simulink model "TransmissionPlant"  (R2026a)
settings: Solver=daessc
libraries: sdl_lib x24, fl_lib x19, nesl_utility x15
(part 2 of 2)

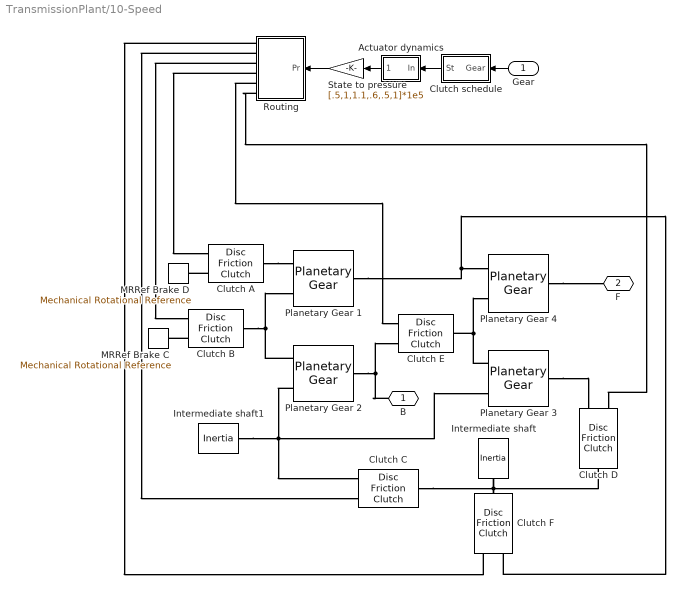
== system TransmissionPlant/10-Speed ==
  Gear : Inport
  Actuator dynamics : Subsystem  mask(First-order lag supporting vector signals){b=[1 1 1 1 1 1]*0.05, x_initial=ClutchSchedule{InitGear}}
      mask prompts: b "Filter time constant"; x_initial "Initial output"
      mask help: Models a lag of the form 1/(b*s+1) where s is the Laplace operator.
  Clutch schedule : Subsystem
  Clutch A : sdl_lib/Clutches/Disc Friction Clutch  geometry_model=1  r_eff=130 mm  d_o=150 mm  d_i=100 mm  nS=6  piston_area=1 m^2  unidirectional=0  friction_model=1  mu_w_vector=[0, 100, 1000] rad/s  temperature_TLU=[280, 300, 320] K  mu_static=0.35  mu_static_vector=[.4, .38, .36]  mu_coulomb=0.3  mu_coulomb_vector=[.3, .22, .19]  mu_coulomb_temp_vector=[.3, .28, .25]  mu_coulomb_matrix=[.34, .32, .3; .3, .28, .25; .25, .2, .15]  mu_interp_method=simscape.enum.interpolation.linear  mu_extrap_method=simscape.enum.extrapolation.linear  d_f=1  w_tol=0.001 rad/s  pressure_min=100 Pa  mu_visc=0 N*m/(rad/s)  initial_state_locked=1  thermal_mass=25 kJ/K  T_init=300 K
  Clutch B : sdl_lib/Clutches/Disc Friction Clutch  geometry_model=1  r_eff=130 mm  d_o=150 mm  d_i=100 mm  nS=10  piston_area=1 m^2  unidirectional=0  friction_model=1  mu_w_vector=[0, 100, 1000] rad/s  temperature_TLU=[280, 300, 320] K  mu_static=0.35  mu_static_vector=[.4, .38, .36]  mu_coulomb=0.3  mu_coulomb_vector=[.3, .22, .19]  mu_coulomb_temp_vector=[.3, .28, .25]  mu_coulomb_matrix=[.34, .32, .3; .3, .28, .25; .25, .2, .15]  mu_interp_method=simscape.enum.interpolation.linear  mu_extrap_method=simscape.enum.extrapolation.linear  d_f=1  w_tol=0.001 rad/s  pressure_min=100 Pa  mu_visc=0 N*m/(rad/s)  initial_state_locked=1  thermal_mass=25 kJ/K  T_init=300 K
  Clutch C : sdl_lib/Clutches/Disc Friction Clutch  geometry_model=1  r_eff=130 mm  d_o=150 mm  d_i=100 mm  nS=10  piston_area=1 m^2  unidirectional=0  friction_model=1  mu_w_vector=[0, 100, 1000] rad/s  temperature_TLU=[280, 300, 320] K  mu_static=0.35  mu_static_vector=[.4, .38, .36]  mu_coulomb=0.3  mu_coulomb_vector=[.3, .22, .19]  mu_coulomb_temp_vector=[.3, .28, .25]  mu_coulomb_matrix=[.34, .32, .3; .3, .28, .25; .25, .2, .15]  mu_interp_method=simscape.enum.interpolation.linear  mu_extrap_method=simscape.enum.extrapolation.linear  d_f=1  w_tol=0.001 rad/s  pressure_min=100 Pa  mu_visc=0 N*m/(rad/s)  initial_state_locked=0  thermal_mass=25 kJ/K  T_init=300 K
  Clutch D : sdl_lib/Clutches/Disc Friction Clutch  geometry_model=1  r_eff=130 mm  d_o=150 mm  d_i=100 mm  nS=12  piston_area=1 m^2  unidirectional=0  friction_model=1  mu_w_vector=[0, 100, 1000] rad/s  temperature_TLU=[280, 300, 320] K  mu_static=0.35  mu_static_vector=[.4, .38, .36]  mu_coulomb=0.3  mu_coulomb_vector=[.3, .22, .19]  mu_coulomb_temp_vector=[.3, .28, .25]  mu_coulomb_matrix=[.34, .32, .3; .3, .28, .25; .25, .2, .15]  mu_interp_method=simscape.enum.interpolation.linear  mu_extrap_method=simscape.enum.extrapolation.linear  d_f=1  w_tol=0.001 rad/s  pressure_min=100 Pa  mu_visc=0 N*m/(rad/s)  initial_state_locked=1  thermal_mass=25 kJ/K  T_init=300 K
  Clutch E : sdl_lib/Clutches/Disc Friction Clutch  geometry_model=1  r_eff=130 mm  d_o=150 mm  d_i=100 mm  nS=10  piston_area=1 m^2  unidirectional=0  friction_model=1  mu_w_vector=[0, 100, 1000] rad/s  temperature_TLU=[280, 300, 320] K  mu_static=0.35  mu_static_vector=[.4, .38, .36]  mu_coulomb=0.3  mu_coulomb_vector=[.3, .22, .19]  mu_coulomb_temp_vector=[.3, .28, .25]  mu_coulomb_matrix=[.34, .32, .3; .3, .28, .25; .25, .2, .15]  mu_interp_method=simscape.enum.interpolation.linear  mu_extrap_method=simscape.enum.extrapolation.linear  d_f=1  w_tol=0.001 rad/s  pressure_min=100 Pa  mu_visc=0 N*m/(rad/s)  initial_state_locked=0  thermal_mass=25 kJ/K  T_init=300 K
  Clutch F : sdl_lib/Clutches/Disc Friction Clutch  geometry_model=1  r_eff=130 mm  d_o=150 mm  d_i=100 mm  nS=8  piston_area=1 m^2  unidirectional=0  friction_model=1  mu_w_vector=[0, 100, 1000] rad/s  temperature_TLU=[280, 300, 320] K  mu_static=0.35  mu_static_vector=[.4, .38, .36]  mu_coulomb=0.3  mu_coulomb_vector=[.3, .22, .19]  mu_coulomb_temp_vector=[.3, .28, .25]  mu_coulomb_matrix=[.34, .32, .3; .3, .28, .25; .25, .2, .15]  mu_interp_method=simscape.enum.interpolation.linear  mu_extrap_method=simscape.enum.extrapolation.linear  d_f=1  w_tol=0.001 rad/s  pressure_min=100 Pa  mu_visc=0 N*m/(rad/s)  initial_state_locked=0  thermal_mass=25 kJ/K  T_init=300 K
  Intermediate shaft : fl_lib/Mechanical/Rotational Elements/Inertia  inertia=0.01 kg*m^2  num_ports=foundation.enum.numPorts2.one  w_specify=off  w_priority=High  w=0 rad/s  w_nominal_specify=off  w_nominal_value=1  w_nominal_unit=rad/s  t_specify=off  t_priority=High  t=0 N*m  t_nominal_specify=off  t_nominal_value=1  t_nominal_unit=N*m
  Intermediate shaft1 : fl_lib/Mechanical/Rotational Elements/Inertia  inertia=0.01 kg*m^2  num_ports=foundation.enum.numPorts2.one  w_specify=off  w_priority=High  w=0 rad/s  w_nominal_specify=off  w_nominal_value=1  w_nominal_unit=rad/s  t_specify=off  t_priority=High  t=0 N*m  t_nominal_specify=off  t_nominal_value=1  t_nominal_unit=N*m
  MRRef Brake C : fl_lib/Mechanical/Rotational Elements/Mechanical Rotational Reference
  MRRef Brake D : fl_lib/Mechanical/Rotational Elements/Mechanical Rotational Reference
  Planetary Gear 1 : sdl_lib/Gears/Planetary Gear  rs_ratio=92/44  friction_model=1  efficiency=[ 0.96 0.98 ]  temperature_TLU=[ 280 300 320 ] K  efficiency_sp_TLU=[ 0.95 0.9 0.85 ]  efficiency_rp_TLU=[ 0.95 0.9 0.85 ]  pwr_thr=[ 0.001 0.001 ] W  mu_visc=[ 0 0 ] N*m/(rad/s)  model_inertia=0  sun_inertia=1e-10 kg*m^2  ring_inertia=1e-10 kg*m^2  carrier_inertia=1e-10 kg*m^2  carrier_radius=0.01 m  planet_inertia=0.001 kg*m^2  planet_mass=1e-10 kg  thermal_mass=50 J/K  T_init=300 K
  Planetary Gear 2 : sdl_lib/Gears/Planetary Gear  rs_ratio=89/51  friction_model=1  efficiency=[ 0.96 0.98 ]  temperature_TLU=[ 280 300 320 ] K  efficiency_sp_TLU=[ 0.95 0.9 0.85 ]  efficiency_rp_TLU=[ 0.95 0.9 0.85 ]  pwr_thr=[ 0.001 0.001 ] W  mu_visc=[ 0 0 ] N*m/(rad/s)  model_inertia=0  sun_inertia=1e-10 kg*m^2  ring_inertia=1e-10 kg*m^2  carrier_inertia=1e-10 kg*m^2  carrier_radius=0.01 m  planet_inertia=0.001 kg*m^2  planet_mass=1e-10 kg  thermal_mass=50 J/K  T_init=300 K
  Planetary Gear 3 : sdl_lib/Gears/Planetary Gear  rs_ratio=101/63  friction_model=1  efficiency=[ 0.96 0.98 ]  temperature_TLU=[ 280 300 320 ] K  efficiency_sp_TLU=[ 0.95 0.9 0.85 ]  efficiency_rp_TLU=[ 0.95 0.9 0.85 ]  pwr_thr=[ 0.001 0.001 ] W  mu_visc=[ 0 0 ] N*m/(rad/s)  model_inertia=0  sun_inertia=1e-10 kg*m^2  ring_inertia=1e-10 kg*m^2  carrier_inertia=1e-10 kg*m^2  carrier_radius=0.01 m  planet_inertia=0.001 kg*m^2  planet_mass=1e-10 kg  thermal_mass=50 J/K  T_init=300 K
  Planetary Gear 4 : sdl_lib/Gears/Planetary Gear  rs_ratio=85/23  friction_model=1  efficiency=[ 0.96 0.98 ]  temperature_TLU=[ 280 300 320 ] K  efficiency_sp_TLU=[ 0.95 0.9 0.85 ]  efficiency_rp_TLU=[ 0.95 0.9 0.85 ]  pwr_thr=[ 0.001 0.001 ] W  mu_visc=[ 0 0 ] N*m/(rad/s)  model_inertia=0  sun_inertia=1e-10 kg*m^2  ring_inertia=1e-10 kg*m^2  carrier_inertia=1e-10 kg*m^2  carrier_radius=0.01 m  planet_inertia=0.001 kg*m^2  planet_mass=1e-10 kg  thermal_mass=50 J/K  T_init=300 K
  Routing : Subsystem
  State to pressure : Gain  Gain=[.5,1,1.1,.6,.5,1]*1e5
  B : PMIOPort  Side=Left
  F : PMIOPort  Port=2  Side=Right
  wires:
  Gear/1 -> Clutch schedule/1(Gear)
  Clutch schedule/1(St) -> Actuator dynamics/1(In)
  State to pressure/1 -> Routing/1(Pr)
  Actuator dynamics/1(Out) -> State to pressure/1
  connections:
  Clutch A/LConn2 -- MRRef Brake D/LConn1
  Clutch B/LConn2 -- MRRef Brake C/LConn1
  Planetary Gear 4/LConn1 -- F/RConn1
  B/RConn1 -- Planetary Gear 2/LConn1 -- Clutch E/LConn2
  Clutch A/RConn1 -- Planetary Gear 1/RConn1
  Clutch B/RConn1 -- Planetary Gear 1/RConn2 -- Planetary Gear 2/RConn2
  Planetary Gear 1/LConn1 -- Planetary Gear 4/RConn1 -- Clutch F/LConn2
  Planetary Gear 2/RConn1 -- Intermediate shaft1/LConn1 -- Planetary Gear 3/RConn2 -- Clutch C/LConn2
  Planetary Gear 3/RConn1 -- Clutch E/RConn1 -- Planetary Gear 4/RConn2
  Planetary Gear 3/LConn1 -- Clutch D/LConn2
  Clutch F/RConn1 -- Clutch C/RConn1 -- Intermediate shaft/LConn1 -- Clutch D/RConn1
  Routing/RConn1 -- Clutch F/LConn1
  Routing/RConn2 -- Clutch C/LConn1
  Routing/RConn3 -- Clutch B/LConn1
  Routing/RConn4 -- Clutch A/LConn1
  Routing/RConn5 -- Clutch E/LConn1
  Routing/RConn6 -- Clutch D/LConn1

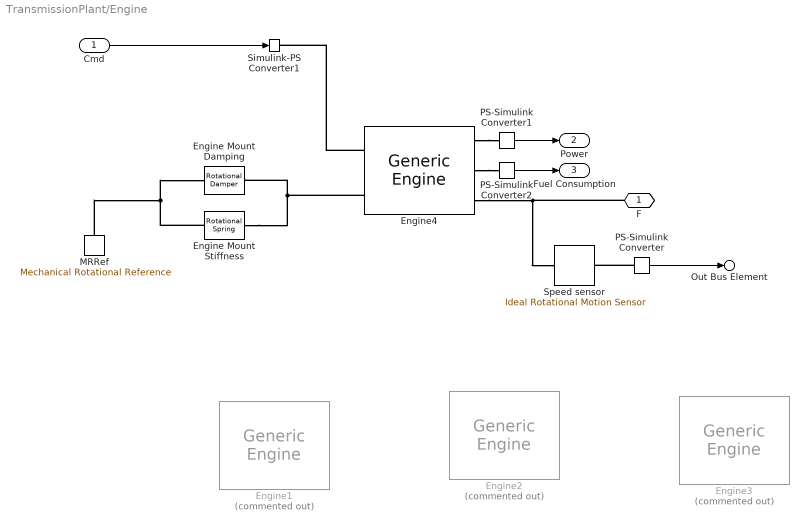
== system TransmissionPlant/Engine ==
  Cmd : Inport
  Engine Mount Damping : fl_lib/Mechanical/Rotational Elements/Rotational Damper  D=10000 N*m/rpm  w_specify=on  w_priority=High  w=0 rad/s  w_nominal_specify=off  w_nominal_value=1  w_nominal_unit=rad/s  t_specify=off  t_priority=High  t=0 N*m  t_nominal_specify=off  t_nominal_value=1  t_nominal_unit=N*m
      settings: AttributesFormatString=|
      | %<D>
      | %<D_unit>
  Engine Mount Stiffness : fl_lib/Mechanical/Rotational Elements/Rotational Spring  spr_rate=10 N*m/rad  w_specify=on  w_priority=High  w=0 rad/s  w_nominal_specify=off  w_nominal_value=1  w_nominal_unit=rad/s  t_specify=off  t_priority=High  t=0 N*m  t_nominal_specify=off  t_nominal_value=1  t_nominal_unit=N*m  phi_specify=off  phi_priority=High  phi=0 rad  phi_nominal_specify=off  phi_nominal_value=1  phi_nominal_unit=rad
      settings: AttributesFormatString=|
      | %<spr_rate>
      | %<spr_rate_unit>
  Engine1 : sdl_lib/Engines & Motors/Generic Engine  Commented=on  input_type=sdl.enum.GenericEngineInputType.NormalizedThrottle  model_parameterization=1  engine_type=1  Trq_max=380 N*m  w_Trq_max=4300 rpm  P_max=100 kW  w_P_max=5500 rpm  w_max=7500 rpm  w_min=200 rpm  w_tab=[ 500 1000 2e+3 3e+3 4e+3 5e+3 6e+3 7e+3 ] rpm  trq_tab=[ 380 380 380 380 350 280 200 80 ] N*m  pwr_tab=[ 2e+4 4e+4 7.8e+4 1.2e+5 1.45e+5 1.48e+5 1.25e+5 6e+4 ] W  interp_method=simscape.enum.interpolation.linear  w_thr=20 rpm  model_inertia=1  inertia=0.2 kg*m^2  initial_velocity=800 rpm  model_time_constant=1  time_constant=0.2 s  initial_normalized_throttle=0  fc_model=sdl.enum.fuel_consumption_model.FuelSpeedTorque  fc_per_rev=25 mg/rev  fc_w_tab=[ 1000 2e+3 3e+3 4e+3 5e+3 6e+3 ] rpm  fc_trq_tab=[ 0 80 160 200 240 320 360 400 ] N*m  fc_tab=[ 0.5 0.9 1.4 1.6 1.9 2.7 3.4 4.4; 1 1.7 2.7 3.1 3.6 5 6 7.4; 1.4 2.7 4 4.8 5.6 7.5 8.5 10.5; 2 3.6 5.8 6.7 8 10.4 11.7 13.3; 2.5 4.8 7.9 9.4 10.8 14 16.2 18.6; 3.1 6 10.3 11.9 13.8 18.4 22 26.5 ] g/s  bmep_tab=[ 0 250 500 625 750 1000 1.15e+3 1.25e+3 ] kPa  bsfc_tab=[ 410 380 300 280 270 290 320 380; 410 370 290 270 260 270 285 320; 415 380 290 275 265 270 270 300; 420 390 310 290 285 280 280 285; 430 410 340 320 310 300 310 320; 450 430 370 340 330 330 350 380 ] g/hr/kW  fc_interp_method=simscape.enum.interpolation.linear  displaced_volume=400 cm^3  rev_per_cycle=2  idle_speed=1  idle_speed_reference=800 rpm  tau_controller=0.1 s  idle_w_thr=1 rpm  redline=true  redline_speed=6800 rpm  tau_redline=1 s  redline_w_thr=1 rpm
      settings: AttributesFormatString=%<initial_velocity> [%<initial_velocity_unit>]
  Engine2 : sdl_lib/Engines & Motors/Generic Engine  Commented=on  PartSpecification="{\"CollectionId\":\"MW.SimscapeDriveline\",\"CollectionVersion\":\"1.0.0\",\"DatasetId\":\"Generic Engine|325 hp Engine Gasoline: Tier 3|simscape.driveline.genericEngine\",\"DisplayName\":\"Generic Engine:325 hp Engine Gasoline: Tier 3\"}"  input_type=sdl.enum.GenericEngineInputType.NormalizedThrottle  model_parameterization=sdl.enum.engineParameterization.torque  engine_type=sdl.enum.engineType.SI  Trq_max=380 % Parameter not set N*m  w_Trq_max=4300 % Parameter not set rpm  P_max=230 % Parameter not set kW  w_P_max=6858 % Parameter not set rpm  w_max=7000 % Parameter not set rpm  w_min=500 % Parameter not set rpm  w_tab=[1000;1501;1751;2000;3000;4250;5750;6037.5] % From weblink database rpm  trq_tab=[230.06;350.03;416.41;460.978;508.432;488.094;402.678;345.153] % From weblink database N*m  pwr_tab=[10, 30, 70, 110, 165, 190, 220, 230] % Parameter not set kW  interp_method=simscape.enum.interpolation.smooth  w_thr=100 % Library default rpm  model_inertia=sdl.enum.model_inertia.off  inertia=1 % Parameter not set kg*m^2  initial_velocity=800 % Parameter not set rpm  model_time_constant=sdl.enum.lagOffOn.off  time_constant=0.2 % Parameter not set s  initial_normalized_throttle=0 % Parameter not set  fc_model=sdl.enum.fuel_consumption_model.FuelSpeedTorque  fc_per_rev=25 % Parameter not set mg/rev  fc_w_tab=[0.01 300.417 600.833 1001.167 1251.115 1501.094 1751.059 2001.1 2251.118 2501.029 2751 3001.972 3502.245 4002.16 4501.969 5013.389 5496.816 5910.908 6325] % From weblink database rpm  fc_trq_tab=[25.219 55.538 80.156 104.375 117.652 144.49 178.614 199.144 225.9 250.615 280.405 315.274 344.012 376.651 405.257 438.688 469.19 491.928 512.891 533.853] % From weblink database N*m  fc_tab=[0.083 0.07 0.099 0.157 0.197 0.294 0.465 0.581 0.733 0.847 0.927 0.915 0.823 0.662 0.507 0.317 0.121 0.01 0.01 0.01;0.144 0.182 0.268 0.356 0.409 0.537 0.747 0.892 1.089 1.26 1.418 1.476 1.444 1.371 1.318 1.284 1.271 1.268 1.268 1.269;0.204 0.297 0.439 0.553 0.622 0.781 1.033 1.206 1.442 1.669 1.906 2.033 2.063 2.084 2.133 2.25 2.42 2.575 2.731 2.893;0.315 0.474 0.631 0.815 0.915 1.114 1.432 1.638 1.907 2.189 2.536 2.752 2.885 3.058 3.239 3.532 3.942 4.313 4.682 5.062;0.375 0.605 0.801 1.005 1.111 1.33 1.704 1.914 2.212 2.49 2.88 3.17 3.403 3.693 3.955 4.329 4.887 5.397 5.901 6.416;0.442 0.725 0.966 1.194 1.319 1.58 1.955 2.18 2.463 2.767 3.161 3.565 3.929 4.346 4.69 5.13 5.833 6.482 7.117 7.764;0.515 0.865 1.126 1.387 1.538 1.836 2.226 2.459 2.751 3.077 3.467 3.973 4.474 5.016 5.445 5.95 6.788 7.569 8.326 9.099;0.614 1.009 1.279 1.58 1.753 2.095 2.514 2.765 3.093 3.436 3.845 4.405 5.024 5.695 6.204 6.831 7.765 8.656 9.521 10.407;0.729 1.156 1.455 1.794 1.985 2.366 2.819 3.098 3.472 3.839 4.275 4.847 5.521 6.331 6.961 7.851 8.794 9.729 10.689 11.668;0.844 1.301 1.643 2.025 2.235 2.649 3.138 3.447 3.868 4.27 4.727 5.336 6.061 6.939 7.634 8.773 9.686 10.759 11.821 12.857;0.974 1.456 1.844 2.26 2.487 2.936 3.473 3.813 4.27 4.71 5.197 5.865 6.557 7.562 8.42 9.477 10.34 11.729 12.888 13.941;1.116 1.631 2.065 2.5 2.742 3.231 3.827 4.193 4.675 5.132 5.67 6.4 7.135 8.235 9.263 9.923 10.776 12.604 13.823 14.901;1.348 1.962 2.472 2.982 3.265 3.844 4.568 4.99 5.494 5.982 6.627 7.523 8.433 9.572 10.47 11.259 12.038 12.938 14.583 16.301;1.581 2.321 2.919 3.492 3.809 4.475 5.31 5.762 6.337 6.921 7.762 8.873 9.933 11.065 11.831 13.006 14.082 15.187 16.454 17.83;1.909 2.716 3.377 4.035 4.397 5.139 6.086 6.635 7.339 8.038 9.13 10.479 11.735 13.201 14.563 16.257 17.398 18.298 19.183 20.103;2.232 3.084 3.824 4.577 4.997 5.859 7.005 7.727 8.714 9.714 11.061 12.755 14.229 16.286 18.734 20.266 21.207 21.896 22.545 23.203;2.48 3.426 4.246 5.096 5.576 6.581 7.98 8.9 10.19 11.491 13.205 15.377 17.023 19.824 22.002 23.679 24.736 25.425 26.039 26.647;2.653 3.705 4.608 5.548 6.084 7.222 8.859 9.957 11.505 13.063 15.092 17.629 19.777 22.493 24.574 26.43 27.67 28.454 29.131 29.794;2.811 3.977 4.968 6.003 6.598 7.873 9.753 11.029 12.833 14.646 17.001 19.966 22.462 25.107 27.137 29.13 30.565 31.475 32.251 33.004] % From weblink database g/s  bmep_tab=[0, 250, 500, 625, 750, 1000, 1150, 1250] % Parameter not set kPa  bsfc_tab=[410, 380, 300, 280, 270, 290, 320, 380; 410, 370, 290, 270, 260, 270, 285, 320; 415, 380, 290, 275, 265, 270, 270, 300; 420, 390, 310, 290, 285, 280, 280, 285; 430, 410, 340, 320, 310, 300, 310, 320; 450, 430, 370, 340, 330, 330, 350, 380] % Parameter not set g/(hr*kW)  fc_interp_method=simscape.enum.interpolation.linear  displaced_volume=400 % Parameter not set cm^3  rev_per_cycle=2 % Parameter not set  idle_speed=true  idle_speed_reference=800 rpm  tau_controller=0.1 s  idle_w_thr=1 rpm  redline=true  redline_speed=5000 % Parameter not set rpm  tau_redline=0.1 s  redline_w_thr=1 % Parameter not set rpm
      settings: AttributesFormatString=Generic Engine:325 hp Engine Gasoline: Tier 3
  Engine3 : sdl_lib/Engines & Motors/Generic Engine  Commented=on  PartSpecification="{\"CollectionId\":\"MW.SimscapeDriveline\",\"CollectionVersion\":\"1.0.0\",\"DatasetId\":\"Generic Engine|155 hp Engine Gasoline: Tier 2|simscape.driveline.genericEngine\",\"DisplayName\":\"Generic Engine:155 hp Engine Gasoline: Tier 2\"}"  input_type=sdl.enum.GenericEngineInputType.NormalizedThrottle  model_parameterization=sdl.enum.engineParameterization.polynomial  engine_type=sdl.enum.engineType.SI  Trq_max=380 % Parameter not set N*m  w_Trq_max=4300 % Parameter not set rpm  P_max=230 % Parameter not set kW  w_P_max=6858 % Parameter not set rpm  w_max=7000 % Parameter not set rpm  w_min=500 % Parameter not set rpm  w_tab=[1012.176;1202.696;1301.407;1499.571;1699.486;1900.487;2000.333;2199.867;2400.438;2700.87;2997.792;3300.957;3400.557;3801.205;4100.143;4482.885;6000;6250;6562.5] % From weblink database rpm  trq_tab=[138.688;150.113;153.022;164.067;167.811;183.362;187.874;188.469;182.602;188.231;201.838;199.89;197.399;196.929;200.098;195.305;184;160;130] % From weblink database N*m  pwr_tab=[10, 30, 70, 110, 165, 190, 220, 230] % Parameter not set kW  interp_method=simscape.enum.interpolation.smooth  w_thr=100 % Library default rpm  model_inertia=sdl.enum.model_inertia.off  inertia=1 % Parameter not set kg*m^2  initial_velocity=800 % Parameter not set rpm  model_time_constant=sdl.enum.lagOffOn.off  time_constant=0.2 % Parameter not set s  initial_normalized_throttle=0 % Parameter not set  fc_model=sdl.enum.fuel_consumption_model.FuelSpeedTorque  fc_per_rev=25 % Parameter not set mg/rev  fc_w_tab=[0.01 370.5 741.001 847.204 987.232 1249.539 1497.588 1640.802 1746.865 1869.12 1998.314 2495.794 2995.594 3494.811 3994.431 4494.065 4997.033 5500 6187.5 6875] % From weblink database rpm  fc_trq_tab=[0.519 9.925 19.919 29.858 39.992 49.571 59.937 69.931 80.019 89.98 99.967 110.094 119.924 129.762 139.529 150.227 160.094 169.961 181.674 188.912 196.15 204.039 211.929] % From weblink database N*m  fc_tab=[0.03 0.049 0.069 0.084 0.09 0.088 0.083 0.08 0.082 0.091 0.108 0.135 0.175 0.232 0.304 0.393 0.472 0.547 0.629 0.678 0.725 0.775 0.825;0.074 0.096 0.13 0.168 0.186 0.202 0.219 0.238 0.262 0.292 0.33 0.379 0.435 0.503 0.588 0.699 0.806 0.91 1.033 1.107 1.181 1.262 1.343;0.12 0.145 0.192 0.247 0.28 0.316 0.356 0.396 0.44 0.494 0.552 0.621 0.698 0.778 0.874 1.001 1.135 1.274 1.436 1.536 1.637 1.749 1.863;0.133 0.161 0.211 0.267 0.307 0.349 0.395 0.441 0.492 0.551 0.616 0.69 0.775 0.86 0.957 1.086 1.228 1.379 1.551 1.659 1.768 1.889 2.012;0.15 0.184 0.239 0.295 0.344 0.392 0.447 0.502 0.56 0.627 0.7 0.781 0.876 0.968 1.067 1.197 1.349 1.517 1.704 1.82 1.94 2.073 2.208;0.185 0.234 0.296 0.358 0.425 0.479 0.549 0.615 0.689 0.766 0.859 0.951 1.063 1.177 1.278 1.403 1.572 1.774 1.987 2.124 2.264 2.42 2.576;0.219 0.283 0.355 0.43 0.503 0.574 0.66 0.738 0.824 0.913 1.008 1.108 1.23 1.39 1.488 1.6 1.775 2.002 2.254 2.414 2.574 2.748 2.921;0.241 0.312 0.392 0.472 0.55 0.63 0.72 0.811 0.904 1.002 1.099 1.2 1.321 1.486 1.601 1.72 1.892 2.121 2.409 2.584 2.755 2.938 3.119;0.257 0.333 0.419 0.504 0.586 0.671 0.764 0.865 0.964 1.069 1.169 1.269 1.389 1.552 1.679 1.809 1.979 2.202 2.524 2.711 2.89 3.079 3.265;0.276 0.357 0.451 0.54 0.628 0.718 0.814 0.926 1.035 1.147 1.251 1.352 1.468 1.624 1.763 1.91 2.08 2.288 2.657 2.858 3.046 3.241 3.432;0.297 0.382 0.484 0.577 0.672 0.769 0.867 0.991 1.109 1.229 1.34 1.441 1.555 1.702 1.849 2.017 2.189 2.378 2.802 3.016 3.212 3.413 3.609;0.377 0.483 0.598 0.717 0.844 0.971 1.116 1.253 1.396 1.543 1.69 1.831 1.983 2.11 2.269 2.454 2.679 2.993 3.49 3.68 3.862 4.068 4.281;0.483 0.6 0.733 0.878 1.034 1.195 1.371 1.538 1.706 1.869 2.031 2.217 2.39 2.561 2.732 2.935 3.186 3.519 4.011 4.272 4.506 4.764 5.013;0.579 0.725 0.888 1.074 1.271 1.456 1.646 1.845 2.041 2.234 2.438 2.651 2.861 3.047 3.228 3.44 3.687 4.019 4.608 4.978 5.291 5.565 5.835;0.718 0.885 1.077 1.302 1.55 1.758 1.989 2.19 2.396 2.612 2.838 3.077 3.311 3.538 3.765 4.002 4.277 4.651 5.258 5.633 5.992 6.399 6.838;0.852 1.067 1.296 1.52 1.753 2.009 2.282 2.537 2.784 3.024 3.262 3.525 3.779 4.029 4.294 4.637 4.998 5.427 6.205 6.684 7.15 7.648 8.145;1.017 1.263 1.52 1.77 2.031 2.296 2.598 2.896 3.197 3.49 3.771 4.042 4.303 4.584 4.919 5.406 5.996 6.692 7.594 8.118 8.619 9.148 9.669;1.185 1.463 1.755 2.029 2.314 2.597 2.923 3.257 3.608 3.964 4.312 4.608 4.903 5.241 5.654 6.269 7.123 8.094 9.198 9.724 10.223 10.765 11.309;1.401 1.709 2.034 2.354 2.683 3.003 3.365 3.734 4.126 4.527 4.939 5.373 5.833 6.366 7.002 7.855 8.784 9.786 10.969 11.655 12.316 13.016 13.709;1.604 1.946 2.308 2.668 3.037 3.391 3.786 4.184 4.613 5.075 5.591 6.186 6.846 7.595 8.426 9.43 10.423 11.462 12.742 13.545 14.352 15.232 16.112] % From weblink database g/s  bmep_tab=[0, 250, 500, 625, 750, 1000, 1150, 1250] % Parameter not set kPa  bsfc_tab=[410, 380, 300, 280, 270, 290, 320, 380; 410, 370, 290, 270, 260, 270, 285, 320; 415, 380, 290, 275, 265, 270, 270, 300; 420, 390, 310, 290, 285, 280, 280, 285; 430, 410, 340, 320, 310, 300, 310, 320; 450, 430, 370, 340, 330, 330, 350, 380] % Parameter not set g/(hr*kW)  fc_interp_method=simscape.enum.interpolation.linear  displaced_volume=400 % Parameter not set cm^3  rev_per_cycle=2 % Parameter not set  idle_speed=true  idle_speed_reference=1000 % Parameter not set rpm  tau_controller=1 % Parameter not set s  idle_w_thr=1 % Parameter not set rpm  redline=true  redline_speed=5000 % Parameter not set rpm  tau_redline=1 % Parameter not set s  redline_w_thr=1 % Parameter not set rpm
      settings: AttributesFormatString=Generic Engine:155 hp Engine Gasoline: Tier 2
  Engine4 : sdl_lib/Engines & Motors/Generic Engine  input_type=sdl.enum.GenericEngineInputType.NormalizedThrottle  model_parameterization=1  engine_type=1  Trq_max=380 N*m  w_Trq_max=4300 rpm  P_max=100 kW  w_P_max=5500 rpm  w_max=7500 rpm  w_min=200 rpm  w_tab=[ 500 1000 2e+3 3e+3 4e+3 5e+3 6e+3 7e+3 ] rpm  trq_tab=[ 380 380 380 380 350 280 200 80 ] N*m  pwr_tab=[ 2e+4 4e+4 7.8e+4 1.2e+5 1.45e+5 1.48e+5 1.25e+5 6e+4 ] W  interp_method=simscape.enum.interpolation.linear  w_thr=20 rpm  model_inertia=1  inertia=0.2 kg*m^2  initial_velocity=800 rpm  model_time_constant=1  time_constant=0.2 s  initial_normalized_throttle=0  fc_model=sdl.enum.fuel_consumption_model.FuelSpeedTorque  fc_per_rev=25 mg/rev  fc_w_tab=[ 1000 2e+3 3e+3 4e+3 5e+3 6e+3 ] rpm  fc_trq_tab=[ 0 80 160 200 240 320 360 400 ] N*m  fc_tab=[ 0.5 0.9 1.4 1.6 1.9 2.7 3.4 4.4; 1 1.7 2.7 3.1 3.6 5 6 7.4; 1.4 2.7 4 4.8 5.6 7.5 8.5 10.5; 2 3.6 5.8 6.7 8 10.4 11.7 13.3; 2.5 4.8 7.9 9.4 10.8 14 16.2 18.6; 3.1 6 10.3 11.9 13.8 18.4 22 26.5 ] g/s  bmep_tab=[ 0 250 500 625 750 1000 1.15e+3 1.25e+3 ] kPa  bsfc_tab=[ 410 380 300 280 270 290 320 380; 410 370 290 270 260 270 285 320; 415 380 290 275 265 270 270 300; 420 390 310 290 285 280 280 285; 430 410 340 320 310 300 310 320; 450 430 370 340 330 330 350 380 ] g/hr/kW  fc_interp_method=simscape.enum.interpolation.linear  displaced_volume=400 cm^3  rev_per_cycle=2  idle_speed=false  idle_speed_reference=800 rpm  tau_controller=0.1 s  idle_w_thr=1 rpm  redline=false  redline_speed=6800 rpm  tau_redline=1 s  redline_w_thr=1 rpm
      settings: AttributesFormatString=%<initial_velocity> [%<initial_velocity_unit>]
  MRRef : fl_lib/Mechanical/Rotational Elements/Mechanical Rotational Reference
  PS-Simulink Converter : nesl_utility/PS-Simulink Converter  PhysicalDomain=network_engine_domain  SubClassName=ps_output  LeftPortType=input  RightPortType=output  PseudoPeriodic=off  Frequencies=[]  VectorFormat=inherit  Unit=rpm  AffineConversion=off
  PS-Simulink Converter1 : nesl_utility/PS-Simulink Converter  PhysicalDomain=network_engine_domain  SubClassName=ps_output  LeftPortType=input  RightPortType=output  PseudoPeriodic=off  Frequencies=[]  VectorFormat=inherit  Unit=inherit  AffineConversion=off
  PS-Simulink Converter2 : nesl_utility/PS-Simulink Converter  PhysicalDomain=network_engine_domain  SubClassName=ps_output  LeftPortType=input  RightPortType=output  PseudoPeriodic=off  Frequencies=[]  VectorFormat=inherit  Unit=inherit  AffineConversion=off
  Simulink-PS Converter1 : nesl_utility/Simulink-PS Converter  PhysicalDomain=network_engine_domain  SubClassName=ps_input  LeftPortType=input  RightPortType=output  PseudoPeriodic=off  Frequencies=[]  NoiseDistribution=none  NoiseParameters=[]  Unit=1  AffineConversion=off  FilteringAndDerivatives=provide  SimscapeFilterOrder=1  InputFilterTimeConstant=0.001  UdotUserProvided=0
  Speed sensor : fl_lib/Mechanical/Mechanical Sensors/Ideal Rotational Motion Sensor  reference=foundation.enum.MeasurementReference.absolute  acceleration_port=false  velocity_port=true  position_port=false  wrap_angle=simscape.enum.onoff.off  offset=0 rad
  F : PMIOPort  Side=Left
  Out Bus Element : Outport  PortName=Info  Element=EngSpd
  Power : Outport  Port=2
  Fuel Consumption : Outport  Port=3
  wires:
  PS-Simulink Converter/1 -> Out Bus Element/1
  Cmd/1 -> Simulink-PS Converter1/1
  PS-Simulink Converter1/1 -> Power/1
  PS-Simulink Converter2/1 -> Fuel Consumption/1
  connections:
  Engine Mount Stiffness/RConn1 -- Engine4/LConn2 -- Engine Mount Damping/RConn1
  F/RConn1 -- Engine4/RConn3 -- Speed sensor/LConn1
  Engine Mount Stiffness/LConn1 -- MRRef/LConn1 -- Engine Mount Damping/LConn1
  PS-Simulink Converter/LConn1 -- Speed sensor/RConn1
  Engine4/LConn1 -- Simulink-PS Converter1/RConn1
  Engine4/RConn1 -- PS-Simulink Converter1/LConn1
  Engine4/RConn2 -- PS-Simulink Converter2/LConn1

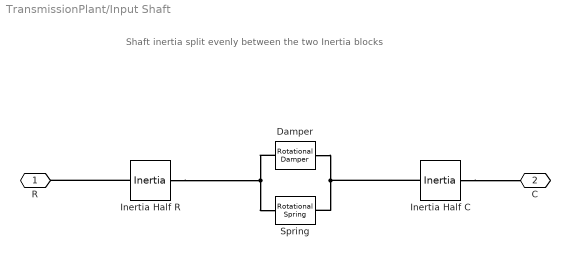
== system TransmissionPlant/Input Shaft ==
  note: Shaft inertia split evenly between the two Inertia blocks
  Damper : fl_lib/Mechanical/Rotational Elements/Rotational Damper  D=10000 N*m/rpm  w_specify=off  w_priority=High  w=0 rad/s  w_nominal_specify=off  w_nominal_value=1  w_nominal_unit=rad/s  t_specify=on  t_priority=High  t=0 N*m  t_nominal_specify=off  t_nominal_value=1  t_nominal_unit=N*m
      settings: AttributesFormatString=|
      | %<D>
      | %<D_unit>
  Inertia Half C : fl_lib/Mechanical/Rotational Elements/Inertia  inertia=0.0015 kg*m^2  num_ports=foundation.enum.numPorts2.two  w_specify=on  w_priority=High  w=800 rpm  w_nominal_specify=off  w_nominal_value=1  w_nominal_unit=rad/s  t_specify=off  t_priority=High  t=0 N*m  t_nominal_specify=off  t_nominal_value=1  t_nominal_unit=N*m
      settings: AttributesFormatString=|
      | %<inertia> %<inertia_unit>
      | %<w> [%<w_unit>]
      | Priority: %<w_priority>
  Inertia Half R : fl_lib/Mechanical/Rotational Elements/Inertia  inertia=0.0015 kg*m^2  num_ports=foundation.enum.numPorts2.two  w_specify=on  w_priority=High  w=800 rpm  w_nominal_specify=off  w_nominal_value=1  w_nominal_unit=rad/s  t_specify=off  t_priority=High  t=0 N*m  t_nominal_specify=off  t_nominal_value=1  t_nominal_unit=N*m
      settings: AttributesFormatString=|
      | %<inertia> %<inertia_unit>
      | %<w> [%<w_unit>]
      | Priority: %<w_priority>
  Spring : fl_lib/Mechanical/Rotational Elements/Rotational Spring  spr_rate=10 N*m/rad  w_specify=off  w_priority=High  w=0 rad/s  w_nominal_specify=off  w_nominal_value=1  w_nominal_unit=rad/s  t_specify=on  t_priority=High  t=0 N*m  t_nominal_specify=off  t_nominal_value=1  t_nominal_unit=N*m  phi_specify=off  phi_priority=High  phi=0 rad  phi_nominal_specify=off  phi_nominal_value=1  phi_nominal_unit=rad
      settings: AttributesFormatString=|
      | %<spr_rate>
      | %<spr_rate_unit>
  R : PMIOPort  Side=Left
  C : PMIOPort  Port=2  Side=Right
  connections:
  Damper/RConn1 -- Inertia Half C/LConn1 -- Spring/RConn1
  Damper/LConn1 -- Inertia Half R/RConn1 -- Spring/LConn1
  Inertia Half C/RConn1 -- C/RConn1
  Inertia Half R/LConn1 -- R/RConn1

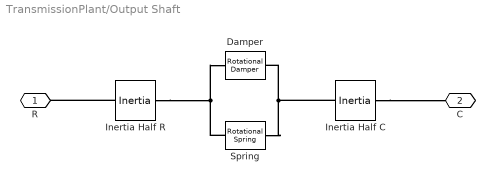
== system TransmissionPlant/Output Shaft ==
  Damper : fl_lib/Mechanical/Rotational Elements/Rotational Damper  D=20000 N*m/rpm  w_specify=off  w_priority=High  w=0 rad/s  w_nominal_specify=off  w_nominal_value=1  w_nominal_unit=rad/s  t_specify=off  t_priority=High  t=0 N*m  t_nominal_specify=off  t_nominal_value=1  t_nominal_unit=N*m
      settings: AttributesFormatString=|
      | %<D>
      | %<D_unit>
  "Inertia Half C " : fl_lib/Mechanical/Rotational Elements/Inertia  inertia=0.0001 kg*m^2  num_ports=foundation.enum.numPorts2.two  w_specify=on  w_priority=High  w=0 rad/s  w_nominal_specify=off  w_nominal_value=1  w_nominal_unit=rad/s  t_specify=off  t_priority=High  t=0 N*m  t_nominal_specify=off  t_nominal_value=1  t_nominal_unit=N*m
      settings: AttributesFormatString=|
      | %<inertia> %<inertia_unit>
      | %<w> [%<w_unit>]
      | Priority: %<w_priority>
  Inertia Half R : fl_lib/Mechanical/Rotational Elements/Inertia  inertia=0.0001 kg*m^2  num_ports=foundation.enum.numPorts2.two  w_specify=on  w_priority=High  w=0 rad/s  w_nominal_specify=off  w_nominal_value=1  w_nominal_unit=rad/s  t_specify=off  t_priority=High  t=0 N*m  t_nominal_specify=off  t_nominal_value=1  t_nominal_unit=N*m
      settings: AttributesFormatString=|
      | %<inertia> %<inertia_unit>
      | %<w> [%<w_unit>]
      | Priority: %<w_priority>
  Spring : fl_lib/Mechanical/Rotational Elements/Rotational Spring  spr_rate=10 N*m/rad  w_specify=off  w_priority=High  w=0 rad/s  w_nominal_specify=off  w_nominal_value=1  w_nominal_unit=rad/s  t_specify=off  t_priority=High  t=0 N*m  t_nominal_specify=off  t_nominal_value=1  t_nominal_unit=N*m  phi_specify=off  phi_priority=High  phi=0 rad  phi_nominal_specify=off  phi_nominal_value=1  phi_nominal_unit=rad
      settings: AttributesFormatString=|
      | %<spr_rate>
      | %<spr_rate_unit>
  R : PMIOPort  Side=Left
  C : PMIOPort  Port=2  Side=Right
  connections:
  Spring/RConn1 -- "Inertia Half C "/LConn1 -- Damper/RConn1
  Spring/LConn1 -- Inertia Half R/RConn1 -- Damper/LConn1
  Inertia Half R/LConn1 -- R/RConn1
  "Inertia Half C "/RConn1 -- C/RConn1

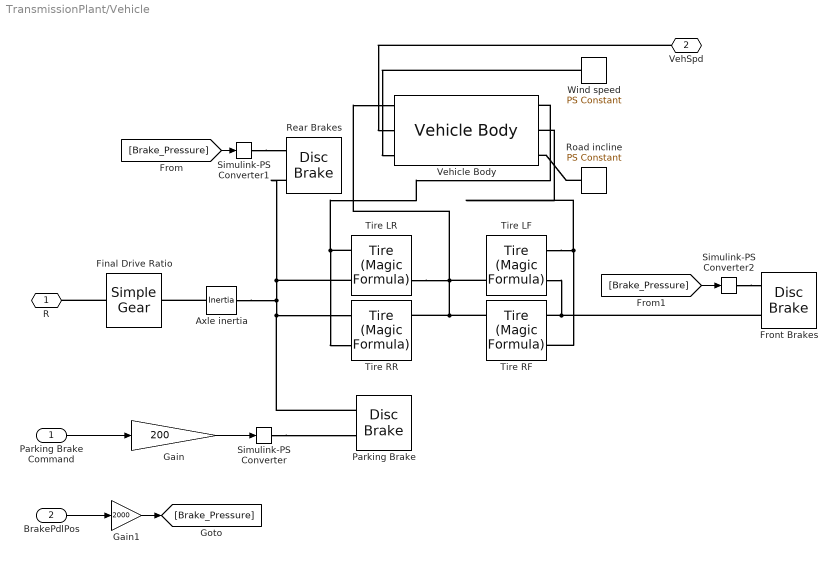
== system TransmissionPlant/Vehicle ==
  Parking Brake Command : Inport
  BrakePdlPos : Inport  Port=2
  Axle inertia : fl_lib/Mechanical/Rotational Elements/Inertia  inertia=0.01 kg*m^2  num_ports=foundation.enum.numPorts2.two  w_specify=on  w_priority=None  w=0 rad/s  w_nominal_specify=off  w_nominal_value=1  w_nominal_unit=rad/s  t_specify=off  t_priority=High  t=0 N*m  t_nominal_specify=off  t_nominal_value=1  t_nominal_unit=N*m
      settings: AttributesFormatString=Priority: %<w_priority>
  Final Drive Ratio : sdl_lib/Gears/Simple Gear  ratio=3.7  rotation_direction=sdl.enum.shaftOutputDirection.same  friction_model=2  T_noload=0.1 N*m  T_nom=5 N*m  efficiency_nom=0.8  efficiency=0.95  temperature_TLU=[ 280 300 320 ] K  load_TLU=[ 1 5 10 ] N*m  efficiency_TLU=[ 0.95 0.9 0.85 ]  efficiency_TLU2=[ 0.85 0.8 0.75; 0.95 0.9 0.85; 0.85 0.8 0.7 ]  w_thr=0.01 rad/s  pwr_thr=1 W  enable_backlash=false  hardstop_model=simscape.enum.hardstop.smooth  backlash_distance=1e-3 mm  r_base=0.1 m  transition=1e-4 mm  backlash_stiffness=1e7 N/m  backlash_damping=1e6 N*s/m  coeff_rest=0  v_tol=0.001 m/s  f_tol=0 N  tau=0.1 s  mu_visc=[0 0] N*m/(rad/s)  thermal_mass=50 J/K  temperature_specify=off  temperature_priority=High  temperature=300 K  temperature_nominal_specify=off  temperature_nominal_value=1  temperature_nominal_unit=K  x_backlash_specify=off  x_backlash_priority=None  x_backlash=0 mm  x_backlash_nominal_specify=off  x_backlash_nominal_value=1  x_backlash_nominal_unit=mm  f_hardstop_specify=off  f_hardstop_priority=None  f_hardstop=0 N  f_hardstop_nominal_specify=off  f_hardstop_nominal_value=1  f_hardstop_nominal_unit=N  v_backlash_specify=off  v_backlash_priority=None  v_backlash=0 m/s  v_backlash_nominal_specify=off  v_backlash_nominal_value=1  v_backlash_nominal_unit=m/s
      settings: AttributesFormatString=Reduction ratio %<ratio>
  Front Brakes : sdl_lib/Brakes & Detents/Rotational/Disc Brake  r_mean=150 mm  bore=10 mm  n_pads=2  thermal_port=simscape.enum.thermaleffects.omit  mu_static=0.9  mu_coulomb=0.7  temperature_TLU=[280, 300, 320] K  mu_static_TLU=[.9, .8, .7]  mu_coulomb_TLU=[.8, .7, .6]  brkwy_vel=0.1 rad/s  visc_coef=0 N*m*s/rad  thermal_mass=50 kJ/K  temperature_specify=off  temperature_priority=High  temperature=300 K  temperature_nominal_specify=off  temperature_nominal_value=1  temperature_nominal_unit=K
  Gain : Gain  Gain=200  OutDataTypeStr=double
  Gain1 : Gain  Gain=2000
  Parking Brake : sdl_lib/Brakes & Detents/Rotational/Disc Brake  r_mean=150 mm  bore=10 mm  n_pads=2  thermal_port=simscape.enum.thermaleffects.omit  mu_static=0.9  mu_coulomb=0.7  temperature_TLU=[280, 300, 320] K  mu_static_TLU=[.9, .8, .7]  mu_coulomb_TLU=[.8, .7, .6]  brkwy_vel=0.1 rad/s  visc_coef=0 N*m*s/rad  thermal_mass=50 kJ/K  temperature_specify=off  temperature_priority=High  temperature=300 K  temperature_nominal_specify=off  temperature_nominal_value=1  temperature_nominal_unit=K
  Rear Brakes : sdl_lib/Brakes & Detents/Rotational/Disc Brake  r_mean=150 mm  bore=10 mm  n_pads=2  thermal_port=simscape.enum.thermaleffects.omit  mu_static=0.9  mu_coulomb=0.7  temperature_TLU=[280, 300, 320] K  mu_static_TLU=[.9, .8, .7]  mu_coulomb_TLU=[.8, .7, .6]  brkwy_vel=0.1 rad/s  visc_coef=0 N*m*s/rad  thermal_mass=50 kJ/K  temperature_specify=off  temperature_priority=High  temperature=300 K  temperature_nominal_specify=off  temperature_nominal_value=1  temperature_nominal_unit=K
  Road incline : fl_lib/Physical Signals/Sources/PS Constant  constant=0
  Simulink-PS Converter : nesl_utility/Simulink-PS Converter  PhysicalDomain=network_engine_domain  SubClassName=ps_input  LeftPortType=input  RightPortType=output  PseudoPeriodic=off  Frequencies=[]  NoiseDistribution=none  NoiseParameters=[]  Unit=1  AffineConversion=off  FilteringAndDerivatives=provide  SimscapeFilterOrder=1  InputFilterTimeConstant=0.001  UdotUserProvided=0
  Simulink-PS Converter1 : nesl_utility/Simulink-PS Converter  PhysicalDomain=network_engine_domain  SubClassName=ps_input  LeftPortType=input  RightPortType=output  PseudoPeriodic=off  Frequencies=[]  NoiseDistribution=none  NoiseParameters=[]  Unit=1  AffineConversion=off  FilteringAndDerivatives=provide  SimscapeFilterOrder=1  InputFilterTimeConstant=0.001  UdotUserProvided=0
  Simulink-PS Converter2 : nesl_utility/Simulink-PS Converter  PhysicalDomain=network_engine_domain  SubClassName=ps_input  LeftPortType=input  RightPortType=output  PseudoPeriodic=off  Frequencies=[]  NoiseDistribution=none  NoiseParameters=[]  Unit=1  AffineConversion=off  FilteringAndDerivatives=provide  SimscapeFilterOrder=1  InputFilterTimeConstant=0.001  UdotUserProvided=0
  Tire LF : sdl_lib/Tires & Vehicles/Tire (Magic Formula)  parameterization=3  F_z1=3000 N  F_x1=3500 N  kappa1=10  B_m=10  C_m=1.9  D_m=1  E_m=0.97  fz0=4000 N  p_Cx=1.685  p_Dx=[ 1.21 -0.037 ]  p_Ex=[ 0.344 0.095 -0.02 0 ]  p_Kx=[ 21.51 -0.163 0.245 ]  p_Hx=[ -0.002 0.002 ]  p_Vx=[ 0 0 ]  rolling_radius_model=sdl.enum.RollingRadiusParameterization.Constant  r_e=0.312 m  r_0=0.3 m  breff=8.39  dreff=0.26  freff=0.074  q_re0=0.99  q_v1=0.008  longvl=17 m/s  cz=5e5 N/m  model_resistance=1  resistance_model=1  coeff=0.015  p_tire=250e3 Pa  alpha=-0.003  beta=0.97  coeff_a=84e-4  coeff_b=6.2e-4 s/m  coeff_c=1.6e-4 s^2/m^2  p_tire0=240e3 Pa  fz0_resistance=4000 N  vH0=16 m/s  q_Sy=[.0082, 0, .0014, .001, 0, 0, 1.08, -.5]  v_thr=1e-3 m/s  enable_scaling_coefficients=false  lfzO=1  lcx=1  lmux=1  lex=1  lkx=1  lhx=1  lvx=1  lmy=1  model_compliance=0  stiffness=1e+6 N/m  damping=1000 N/(m/s)  model_inertia=1  inertia=0.5 kg*m^2  initial_velocity=0 rpm  vxlow=0.1 m/s  v_tr_thr=0.01 m/s  kpumin=-1.5  kpumax=1.5
  Tire LR : sdl_lib/Tires & Vehicles/Tire (Magic Formula)  parameterization=3  F_z1=3000 N  F_x1=3500 N  kappa1=10  B_m=10  C_m=1.9  D_m=1  E_m=0.97  fz0=4000 N  p_Cx=1.685  p_Dx=[ 1.21 -0.037 ]  p_Ex=[ 0.344 0.095 -0.02 0 ]  p_Kx=[ 21.51 -0.163 0.245 ]  p_Hx=[ -0.002 0.002 ]  p_Vx=[ 0 0 ]  rolling_radius_model=sdl.enum.RollingRadiusParameterization.Constant  r_e=0.312 m  r_0=0.3 m  breff=8.39  dreff=0.26  freff=0.074  q_re0=0.99  q_v1=0.008  longvl=17 m/s  cz=5e5 N/m  model_resistance=1  resistance_model=1  coeff=0.015  p_tire=250e3 Pa  alpha=-0.003  beta=0.97  coeff_a=84e-4  coeff_b=6.2e-4 s/m  coeff_c=1.6e-4 s^2/m^2  p_tire0=240e3 Pa  fz0_resistance=4000 N  vH0=16 m/s  q_Sy=[.0082, 0, .0014, .001, 0, 0, 1.08, -.5]  v_thr=1e-3 m/s  enable_scaling_coefficients=false  lfzO=1  lcx=1  lmux=1  lex=1  lkx=1  lhx=1  lvx=1  lmy=1  model_compliance=0  stiffness=1e+6 N/m  damping=1000 N/(m/s)  model_inertia=1  inertia=0.5 kg*m^2  initial_velocity=0 rpm  vxlow=0.1 m/s  v_tr_thr=0.01 m/s  kpumin=-1.5  kpumax=1.5
  Tire RF : sdl_lib/Tires & Vehicles/Tire (Magic Formula)  parameterization=3  F_z1=3000 N  F_x1=3500 N  kappa1=10  B_m=10  C_m=1.9  D_m=1  E_m=0.97  fz0=4000 N  p_Cx=1.685  p_Dx=[ 1.21 -0.037 ]  p_Ex=[ 0.344 0.095 -0.02 0 ]  p_Kx=[ 21.51 -0.163 0.245 ]  p_Hx=[ -0.002 0.002 ]  p_Vx=[ 0 0 ]  rolling_radius_model=sdl.enum.RollingRadiusParameterization.Constant  r_e=0.312 m  r_0=0.3 m  breff=8.39  dreff=0.26  freff=0.074  q_re0=0.99  q_v1=0.008  longvl=17 m/s  cz=5e5 N/m  model_resistance=1  resistance_model=1  coeff=0.015  p_tire=250e3 Pa  alpha=-0.003  beta=0.97  coeff_a=84e-4  coeff_b=6.2e-4 s/m  coeff_c=1.6e-4 s^2/m^2  p_tire0=240e3 Pa  fz0_resistance=4000 N  vH0=16 m/s  q_Sy=[.0082, 0, .0014, .001, 0, 0, 1.08, -.5]  v_thr=1e-3 m/s  enable_scaling_coefficients=false  lfzO=1  lcx=1  lmux=1  lex=1  lkx=1  lhx=1  lvx=1  lmy=1  model_compliance=0  stiffness=1e+6 N/m  damping=1000 N/(m/s)  model_inertia=1  inertia=0.5 kg*m^2  initial_velocity=0 rpm  vxlow=0.1 m/s  v_tr_thr=0.01 m/s  kpumin=-1.5  kpumax=1.5
  Tire RR : sdl_lib/Tires & Vehicles/Tire (Magic Formula)  parameterization=3  F_z1=3000 N  F_x1=3500 N  kappa1=10  B_m=10  C_m=1.9  D_m=1  E_m=0.97  fz0=4000 N  p_Cx=1.685  p_Dx=[ 1.21 -0.037 ]  p_Ex=[ 0.344 0.095 -0.02 0 ]  p_Kx=[ 21.51 -0.163 0.245 ]  p_Hx=[ -0.002 0.002 ]  p_Vx=[ 0 0 ]  rolling_radius_model=sdl.enum.RollingRadiusParameterization.Constant  r_e=0.312 m  r_0=0.3 m  breff=8.39  dreff=0.26  freff=0.074  q_re0=0.99  q_v1=0.008  longvl=17 m/s  cz=5e5 N/m  model_resistance=1  resistance_model=1  coeff=0.015  p_tire=250e3 Pa  alpha=-0.003  beta=0.97  coeff_a=84e-4  coeff_b=6.2e-4 s/m  coeff_c=1.6e-4 s^2/m^2  p_tire0=240e3 Pa  fz0_resistance=4000 N  vH0=16 m/s  q_Sy=[.0082, 0, .0014, .001, 0, 0, 1.08, -.5]  v_thr=1e-3 m/s  enable_scaling_coefficients=false  lfzO=1  lcx=1  lmux=1  lex=1  lkx=1  lhx=1  lvx=1  lmy=1  model_compliance=0  stiffness=1e+6 N/m  damping=1000 N/(m/s)  model_inertia=1  inertia=0.5 kg*m^2  initial_velocity=0 rpm  vxlow=0.1 m/s  v_tr_thr=0.01 m/s  kpumin=-1.5  kpumax=1.5
  Vehicle Body : sdl_lib/Tires & Vehicles/Vehicle Body  mass=1600 kg  n_w=2  x_f=1.7 m  x_r=2 m  y_c=0.5 m  mass_var=simscape.enum.onoff.off  g=9.81 m/s^2  liftoff_warning=0  area=3 m^2  Cd_var=false  Cd=0.4  rho=1.18 kg/m^3  model_pitch=simscape.enum.onoff.on  inertia=4000 kg*m^2  suspension_model=sdl.enum.linearTLU.TLU  k_f=1e4 N/m  b_f=1e4 N/(m/s)  k_r=1e4 N/m  b_r=1e4 N/(m/s)  k_f_TLU=[-2000, -1000, 0, 1000, 2000] N  x_f_TLU=[-.4, -.2, 0, .2, .4] m  b_f_TLU=[-200, -100, 0, 100, 200] N  v_f_TLU=[-4, -2, 0, 2, 4] m/s  k_r_TLU=[-2000, -1000, 0, 1000, 2000] N  x_r_TLU=[-.4, -.2, 0, .2, .4] m  b_r_TLU=[-200, -100, 0, 100, 200] N  v_r_TLU=[-4, -2, 0, 2, 4] m/s  interp_method=simscape.enum.interpolation.linear  extrap_method=simscape.enum.extrapolation.linear  model_hardstop=0  upper_bound_f=.25 m  lower_bound_f=-.25 m  stop_k_f=1e6 N/m  stop_b_f=150 N/(m/s)  upper_bound_r=.25 m  lower_bound_r=-.25 m  stop_k_r=1e6 N/m  stop_b_r=150 N/(m/s)  initial_pitch=0 rad  initial_pitch_rate=0 rad/s  v_specify=on  v_priority=High  v=0 m/s  v_nominal_specify=off  v_nominal_value=1  v_nominal_unit=m/s
  Wind speed : fl_lib/Physical Signals/Sources/PS Constant  constant=5
  R : PMIOPort  Side=Left
  VehSpd : PMIOPort  Port=2  Side=Right
  wires:
  Gain/1 -> Simulink-PS Converter/1
  Parking Brake Command/1 -> Gain/1
  BrakePdlPos/1 -> Gain1/1
  Gain1/1 -> [Brake_Pressure]
  [Brake_Pressure] -> Simulink-PS Converter1/1
  [Brake_Pressure] -> Simulink-PS Converter2/1
  connections:
  Tire RR/RConn2 -- Tire RF/RConn2 -- Tire LR/RConn2 -- Vehicle Body/LConn1 -- Tire LF/RConn2
  Vehicle Body/RConn1 -- Tire LR/LConn1 -- Tire RR/LConn1
  Tire LR/LConn2 -- Axle inertia/LConn1 -- Parking Brake/LConn2 -- Tire RR/LConn2 -- Rear Brakes/LConn2
  Tire RF/LConn1 -- Vehicle Body/RConn2 -- Tire LF/LConn1
  Wind speed/RConn1 -- Vehicle Body/LConn3
  Axle inertia/RConn1 -- Final Drive Ratio/RConn1
  Road incline/RConn1 -- Vehicle Body/RConn3
  Tire LF/LConn2 -- Front Brakes/LConn2 -- Tire RF/LConn2
  Final Drive Ratio/LConn1 -- R/RConn1
  VehSpd/RConn1 -- Vehicle Body/LConn2
  Simulink-PS Converter/RConn1 -- Parking Brake/LConn1
  Simulink-PS Converter1/RConn1 -- Rear Brakes/LConn1
  Simulink-PS Converter2/RConn1 -- Front Brakes/LConn1

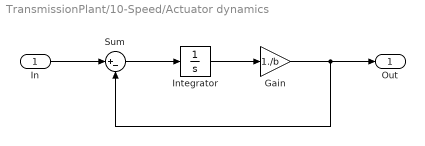
== system TransmissionPlant/10-Speed/Actuator dynamics ==
  In : Inport
  Gain : Gain  Gain=1./b
  Integrator : Integrator  InitialCondition=x_initial.*b
  Sum : Sum  Inputs=|+-  InputSameDT=on  SaturateOnIntegerOverflow=on  OutDataTypeStr=Inherit: Same as first input
  Out : Outport  VectorParamsAs1DForOutWhenUnconnected=off
  wires:
  Gain/1 -> Out/1, Sum/2
  Integrator/1 -> Gain/1
  In/1 -> Sum/1
  Sum/1 -> Integrator/1

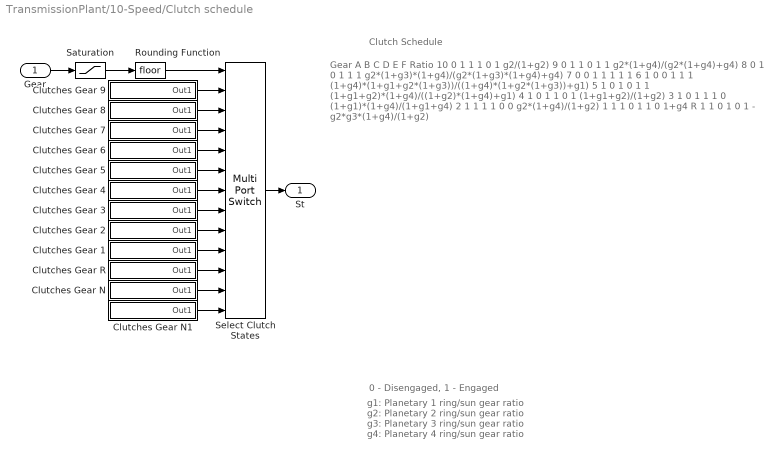
== system TransmissionPlant/10-Speed/Clutch schedule ==
  note: Clutch Schedule
  note: Gear
      | A
      | B
      | C
      | D
      | E
      | F
      | Ratio
      |
      | 10
      | 0
      | 1
      | 1
      | 1
      | 0
      | 1
      | g2/(1+g2)
      |
      | 9
      | 0
      | 1
      | 1
      | 0
      | 1
      | 1
      | g2*(1+g4)/(g2*(1+g4)+g4)
      |
      | 8
      | 0
      | 1
      | 0
      | 1
      | 1
      | 1
      | g2*(1+g3)*(1+g4)/(g2*(1+g3)*(1+g4)+g4)
      |
      | 7
      | 0
      | 0
      | 1
      | 1
      | 1
      | 1
      | 1
      |
      | 6
      | 1
      | 0
      | 0
      | 1
      | 1
      | 1
      | (1+g4)*(1+g1+g2*(1+g3))/((1+g4)*(1+g2*(1+g3))+g1)
      |
      | 5
      | 1
      | 0
      | 1
      | 0
      | 1
      | 1
      | (1+g1+g2)*(1+g4)/((1+g2)*(1+g4)+g1)
      |
      | 4
      | 1
      | 0
      | 1
      | 1
      | 0
      | 1
      | (1+g1+g2)/(1+g2)
      |
      | 3
      | 1
      | 0
      | 1
      | 1
      | 1
      | 0
      | (1+g1)*(1+g4)/(1+g1+g4)
      |
      | 2
      | 1
      | 1
      | 1
      | 1
      | 0
      | 0
      | g2*(1+g4)/(1+g2)
      |
      | 1
      | 1
      | 1
      | 0
      | 1
      | 1
      | 0
      | 1+g4
      |
      | R
      | 1
      | 1
      | 0
      | 1
      | 0
      | 1
      | - g2*g3*(1+g4)/(1+g2)
  note: 0 - Disengaged, 1 - Engaged
  note: g1: Planetary 1 ring/sun gear ratio
      | g2: Planetary 2 ring/sun gear ratio
      | g3: Planetary 3 ring/sun gear ratio
      | g4: Planetary 4 ring/sun gear ratio
  Gear : Inport
  Clutches Gear 1 : Subsystem  mask{Clutches=ClutchSchedule{9}}
      settings: OpenFcn=open_system(gcb,'force');
      mask Display: disp(Clutches)
  Clutches Gear 2 : Subsystem  mask{Clutches=ClutchSchedule{8}}
      settings: OpenFcn=open_system(gcb,'force');
      mask Display: disp(Clutches)
  Clutches Gear 3 : Subsystem  mask{Clutches=ClutchSchedule{7}}
      settings: OpenFcn=open_system(gcb,'force');
      mask Display: disp(Clutches)
  Clutches Gear 4 : Subsystem  mask{Clutches=ClutchSchedule{6}}
      settings: OpenFcn=open_system(gcb,'force');
      mask Display: disp(Clutches)
  Clutches Gear 5 : Subsystem  mask{Clutches=ClutchSchedule{5}}
      settings: OpenFcn=open_system(gcb,'force');
      mask Display: disp(Clutches)
  Clutches Gear 6 : Subsystem  mask{Clutches=ClutchSchedule{4}}
      settings: OpenFcn=open_system(gcb,'force');
      mask Display: disp(Clutches)
  Clutches Gear 7 : Subsystem  mask{Clutches=ClutchSchedule{3}}
      settings: OpenFcn=open_system(gcb,'force');
      mask Display: disp(Clutches)
  Clutches Gear 8 : Subsystem  mask{Clutches=ClutchSchedule{2}}
      settings: OpenFcn=open_system(gcb,'force');
      mask Display: disp(Clutches)
  Clutches Gear 9 : Subsystem  mask{Clutches=ClutchSchedule{1}}
      settings: OpenFcn=open_system(gcb,'force');
      mask Display: disp(Clutches)
  Clutches Gear N : Subsystem  mask{Clutches=ClutchSchedule{11}}
      settings: OpenFcn=open_system(gcb,'force');
      mask Display: disp(Clutches)
  Clutches Gear N1 : Subsystem  mask{Clutches=ClutchSchedule{12}}
      settings: OpenFcn=open_system(gcb,'force');
      mask Display: disp(Clutches)
  Clutches Gear R : Subsystem  mask{Clutches=ClutchSchedule{10}}
      settings: OpenFcn=open_system(gcb,'force');
      mask Display: disp(Clutches)
  Rounding Function : Rounding
  Saturation : Saturate  UpperLimit=10  LowerLimit=-1  ZeroCross=off
  Select Clutch States : MultiPortSwitch  DataPortOrder=Specify indices  DataPortIndices={10,9,8,7,6,5,4,3,2,1,-1,0}  DiagnosticForDefault=None  SaturateOnIntegerOverflow=off  InputSameDT=off
  St : Outport  VectorParamsAs1DForOutWhenUnconnected=off
  wires:
  Select Clutch States/1 -> St/1
  Rounding Function/1 -> Select Clutch States/1
  Saturation/1 -> Rounding Function/1
  Clutches Gear N/1(Out1) -> Select Clutch States/12
  Clutches Gear R/1(Out1) -> Select Clutch States/11
  Clutches Gear 3/1(Out1) -> Select Clutch States/8
  Clutches Gear 2/1(Out1) -> Select Clutch States/9
  Clutches Gear 1/1(Out1) -> Select Clutch States/10
  Clutches Gear 8/1(Out1) -> Select Clutch States/3
  Clutches Gear 5/1(Out1) -> Select Clutch States/6
  Clutches Gear 4/1(Out1) -> Select Clutch States/7
  Clutches Gear 6/1(Out1) -> Select Clutch States/5
  Clutches Gear 7/1(Out1) -> Select Clutch States/4
  Clutches Gear 9/1(Out1) -> Select Clutch States/2
  Gear/1 -> Saturation/1
  Clutches Gear N1/1(Out1) -> Select Clutch States/13

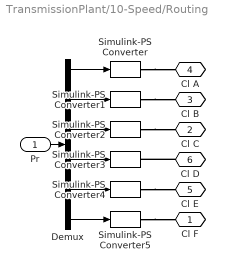
== system TransmissionPlant/10-Speed/Routing ==
  Pr : Inport
  Demux : Demux  Outputs=6
  Simulink-PS Converter{,1..5} (6 alike) : nesl_utility/Simulink-PS Converter  PhysicalDomain=network_engine_domain  SubClassName=ps_input  LeftPortType=input  RightPortType=output  PseudoPeriodic=off  Frequencies=[]  NoiseDistribution=none  NoiseParameters=[]  Unit=1  AffineConversion=off  FilteringAndDerivatives=zero  SimscapeFilterOrder=1  InputFilterTimeConstant=0.001  UdotUserProvided=1
  Cl F : PMIOPort  Side=Right
  Cl C : PMIOPort  Port=2  Side=Right
  Cl B : PMIOPort  Port=3  Side=Right
  Cl A : PMIOPort  Port=4  Side=Right
  Cl E : PMIOPort  Port=5  Side=Right
  Cl D : PMIOPort  Port=6  Side=Right
  wires:
  Demux/6 -> Simulink-PS Converter5/1
  Demux/5 -> Simulink-PS Converter4/1
  Demux/4 -> Simulink-PS Converter3/1
  Demux/3 -> Simulink-PS Converter2/1
  Demux/2 -> Simulink-PS Converter1/1
  Demux/1 -> Simulink-PS Converter/1
  Pr/1 -> Demux/1
  connections:
  Simulink-PS Converter2/RConn1 -- Cl C/RConn1
  Simulink-PS Converter/RConn1 -- Cl A/RConn1
  Simulink-PS Converter1/RConn1 -- Cl B/RConn1
  Cl D/RConn1 -- Simulink-PS Converter3/RConn1
  Simulink-PS Converter4/RConn1 -- Cl E/RConn1
  Simulink-PS Converter5/RConn1 -- Cl F/RConn1

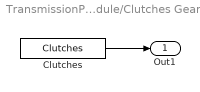
== system TransmissionPlant/10-Speed/Clutch schedule/Clutches Gear 1 ==
  Clutches : Constant  Value=Clutches  SampleTime=0
  Out1 : Outport  VectorParamsAs1DForOutWhenUnconnected=off
  wires:
  Clutches/1 -> Out1/1

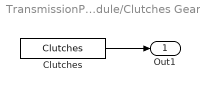
== system TransmissionPlant/10-Speed/Clutch schedule/Clutches Gear 2 ==
  Clutches : Constant  Value=Clutches  SampleTime=0
  Out1 : Outport  VectorParamsAs1DForOutWhenUnconnected=off
  wires:
  Clutches/1 -> Out1/1

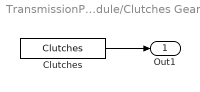
== system TransmissionPlant/10-Speed/Clutch schedule/Clutches Gear 3 ==
  Clutches : Constant  Value=Clutches  SampleTime=0
  Out1 : Outport  VectorParamsAs1DForOutWhenUnconnected=off
  wires:
  Clutches/1 -> Out1/1

== system TransmissionPlant/10-Speed/Clutch schedule/Clutches Gear 4 ==
  Clutches : Constant  Value=Clutches  SampleTime=0
  Out1 : Outport  VectorParamsAs1DForOutWhenUnconnected=off
  wires:
  Clutches/1 -> Out1/1

== system TransmissionPlant/10-Speed/Clutch schedule/Clutches Gear 5 ==
  Clutches : Constant  Value=Clutches  SampleTime=0
  Out1 : Outport  VectorParamsAs1DForOutWhenUnconnected=off
  wires:
  Clutches/1 -> Out1/1

== system TransmissionPlant/10-Speed/Clutch schedule/Clutches Gear 6 ==
  Clutches : Constant  Value=Clutches  SampleTime=0
  Out1 : Outport  VectorParamsAs1DForOutWhenUnconnected=off
  wires:
  Clutches/1 -> Out1/1

== system TransmissionPlant/10-Speed/Clutch schedule/Clutches Gear 7 ==
  Clutches : Constant  Value=Clutches  SampleTime=0
  Out1 : Outport  VectorParamsAs1DForOutWhenUnconnected=off
  wires:
  Clutches/1 -> Out1/1

== system TransmissionPlant/10-Speed/Clutch schedule/Clutches Gear 8 ==
  Clutches : Constant  Value=Clutches  SampleTime=0
  Out1 : Outport  VectorParamsAs1DForOutWhenUnconnected=off
  wires:
  Clutches/1 -> Out1/1

== system TransmissionPlant/10-Speed/Clutch schedule/Clutches Gear 9 ==
  Clutches : Constant  Value=Clutches  SampleTime=0
  Out1 : Outport  VectorParamsAs1DForOutWhenUnconnected=off
  wires:
  Clutches/1 -> Out1/1

== system TransmissionPlant/10-Speed/Clutch schedule/Clutches Gear N ==
  Clutches Gear N : Constant  Value=Clutches  SampleTime=0
  Out1 : Outport  VectorParamsAs1DForOutWhenUnconnected=off
  wires:
  Clutches Gear N/1 -> Out1/1

== system TransmissionPlant/10-Speed/Clutch schedule/Clutches Gear N1 ==
  Clutches Gear N : Constant  Value=Clutches  SampleTime=0
  Out1 : Outport  VectorParamsAs1DForOutWhenUnconnected=off
  wires:
  Clutches Gear N/1 -> Out1/1

== system TransmissionPlant/10-Speed/Clutch schedule/Clutches Gear R ==
  Clutches : Constant  Value=Clutches  SampleTime=0
  Out1 : Outport  VectorParamsAs1DForOutWhenUnconnected=off
  wires:
  Clutches/1 -> Out1/1
